simulink model "a2"  (Simulink 8.7)
settings: Solver=FixedStepAuto  StartTime=0.0  StopTime=0.2  FixedStep=0.005  RelTol=1e-3
settings Model: Creator=birger  LastModifiedBy=birger
settings DataIOCC: LimitDataPoints=off  SaveFormat=Dataset
settings DebuggingCC: UnderspecifiedInitializationDetection=Simplified  MergeDetectMultiDrivingBlocksExec=error
settings HardwareCC: ProdBitPerPointer=64  ProdLargestAtomicFloat=Float  ProdIntDivRoundTo=Zero  ProdEndianess=LittleEndian  ProdWordSize=64  ProdHWDeviceType=Intel->x86-64 (Windows64)
settings ModelReferenceCC: PropagateSignalLabelsOutOfModel=on
settings ConfigComp: CovModelRefEnable=off

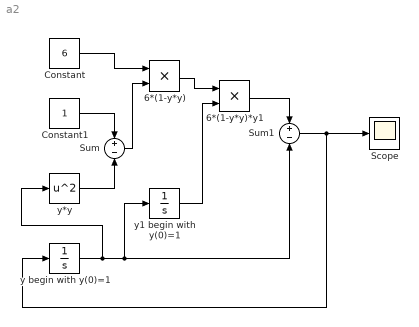
== system a2 ==
  " 6*(1-y*y)" : Product
  6*(1-y*y)*y1 : Product
  Constant : Constant  Value=6
  Constant1 : Constant
  Scope : Scope
  Sum : Sum  Inputs=+-
  Sum1 : Sum  Inputs=+-
  y begin with y(0)=1 : Integrator  InitialCondition=1
  y*y : Math  Operator=square  SaturateOnIntegerOverflow=on
  y1 begin with y(0)=1 : Integrator  InitialCondition=1
  wires:
  Constant/1 -> " 6*(1-y*y)"/1
  Constant1/1 -> Sum/1
  Sum/1 -> " 6*(1-y*y)"/2
  " 6*(1-y*y)"/1 -> 6*(1-y*y)*y1/1
  6*(1-y*y)*y1/1 -> Sum1/1
  Sum1/1 -> Scope/1, y begin with y(0)=1/1
  y*y/1 -> Sum/2
  y begin with y(0)=1/1 -> y1 begin with y(0)=1/1, Sum1/2, y*y/1
  y1 begin with y(0)=1/1 -> 6*(1-y*y)*y1/2
